simulink model "Controller_2_2_BangBang"  (R2019b)
settings: Solver=FixedStepAuto  StartTime=0.0  StopTime=Inf  FixedStep=0.0001  RelTol=1e-3  EnableMultiTasking=on
libraries: arduinolib x5, dspstat3 x2, simulink x1, powerlib_meascontrol x1
settings Model: SILPILModeSetting=veronly  ExtModeTrigDuration=2  Creator=mathe  LastModifiedBy=c3311409
settings OptimizationCC: EnhancedBackFolding=on  PassReuseOutputArgsAs=Individual arguments  ZeroExternalMemoryAtStartup=off  ZeroInternalMemoryAtStartup=off  MaxStackSize=64  OptimizeBlockOrder=speed  DifferentSizesBufferReuse=on  OptimizationCustomize=off  EfficientTunableParamExpr=on
settings DebuggingCC: ParameterTunabilityLossMsg=error
settings HardwareCC: ProdBitPerPointer=32  ProdBitPerSizeT=32  ProdBitPerPtrDiffT=32  ProdLargestAtomicInteger=Long  ProdLargestAtomicFloat=Double  ProdWordSize=32  ProdHWDeviceType=ARM Compatible->ARM Cortex
settings SFSimCC: MATLABDynamicMemAlloc=off
settings RTWCC: SystemTargetFile=ert.tlc  HardwareBoard=Arduino Due  TLCOptions=-aInlineSetEventsForThisBaseRateFcn=TLC_FALSE -aSuppressMultiTaskScheduler=TLC_FALSE -aRateBasedStepFcn=1  TemplateMakefile=ert_default_tmf  GenerateReport=on  Toolchain=Arduino ARM  BuildConfiguration=Faster Runs  IncludeHyperlinkInReport=on  LaunchReport=on  GenerateTraceInfo=on  GenerateTraceReport=on  GenerateTraceReportSl=on  GenerateTraceReportSf=on  GenerateTraceReportEml=on
settings CodeAppCC: ForceParamTrailComments=on  IgnoreCustomStorageClasses=off  OperatorAnnotations=on  SimulinkDataObjDesc=on  SFDataObjDesc=on  InsertBlockDesc=on
settings ERTTargetCC: SupportContinuousTime=on  SupportVariableSizeSignals=on  ExtModeStaticAllocSize=24576

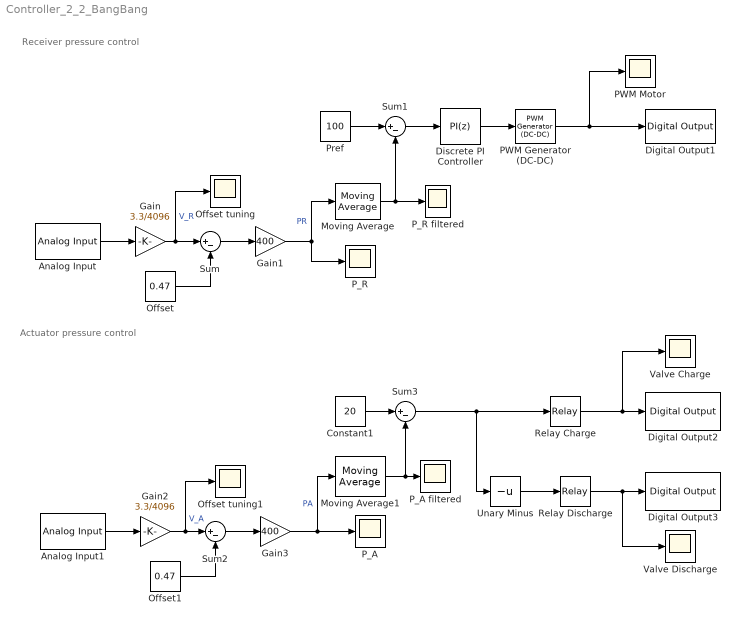
== system Controller_2_2_BangBang ==
  note: Actuator pressure control
  note: Receiver pressure control
  Analog Input : arduinolib/Analog Input  pinNumber=0  ReadResultsOnly=off  ConversionTriggerSource=Software  ExternalTriggerType=uint32(0)  OutputDataType=uint16  EnableConversionCompleteNotify=off  EnableOuputStatus=off  SampleTime=-1  blockPlatform=arduino
  Analog Input1 : arduinolib/Analog Input  pinNumber=1  ReadResultsOnly=off  ConversionTriggerSource=Software  ExternalTriggerType=uint32(0)  OutputDataType=uint16  EnableConversionCompleteNotify=off  EnableOuputStatus=off  SampleTime=-1  blockPlatform=arduino
  Constant1 : Constant  Value=20
  Digital Output1 : arduinolib/Digital Output  pinNumber=7  blockPlatform=arduino
  Digital Output2 : arduinolib/Digital Output  pinNumber=13  blockPlatform=arduino
  Digital Output3 : arduinolib/Digital Output  pinNumber=12  blockPlatform=arduino
  Discrete PI Controller : simulink/Continuous/PID Controller  Controller=PI  Form=Ideal  TimeDomain=Discrete-time  SampleTime=0.0001  IntegratorMethod=Trapezoidal  FilterMethod=Forward Euler  ControllerParametersSource=internal  P=0.001  I=10/(0.005*60)  D=0  UseFilter=on  N=100  TunerSelectOption=Transfer Function Based (PID Tuner App)  InitialConditionSource=internal  InitialConditionForIntegrator=0  InitialConditionForFilter=0  DifferentiatorICPrevScaledInput=0  ExternalReset=none  TrackingMode=off  Kt=1  LimitOutput=on  UpperSaturationLimit=1  LowerSaturationLimit=0  LinearizeAsGain=off  AntiWindupMode=clamping  Kb=1  POutMin=[]  POutMax=[]  IOutMin=[]  IOutMax=[]  DOutMin=[]  DOutMax=[]  NOutMin=[]  NOutMax=[]  SumOutMin=[]  SumOutMax=[]  SaturationOutMin=[]  SaturationOutMax=[]  PParamMin=[]  PParamMax=[]  IParamMin=[]  IParamMax=[]  DParamMin=[]  DParamMax=[]  NParamMin=[]  NParamMax=[]  KbParamMin=[]  KbParamMax=[]  KtParamMin=[]  KtParamMax=[]  KbOutMin=[]  KbOutMax=[]  KtOutMin=[]  KtOutMax=[]  IntegratorOutMin=[]  IntegratorOutMax=[]  FilterOutMin=[]  FilterOutMax=[]  SumI1OutMin=[]  SumI1OutMax=[]  SumI2OutMin=[]  SumI2OutMax=[]  SumI3OutMin=[]  SumI3OutMax=[]  SumI4OutMin=[]  SumI4OutMax=[]  SumDOutMin=[]  SumDOutMax=[]  DifferentiatorOutMin=[]  DifferentiatorOutMax=[]  FilterDiffOutCoefMin=[]  FilterDiffOutCoefMax=[]  ReciprocalOutMin=[]  ReciprocalOutMax=[]  SumDenOutMin=[]  SumDenOutMax=[]  SumNumOutMin=[]  SumNumOutMax=[]  DivideOutMin=[]  DivideOutMax=[]  IntegratorContinuousStateAttributes=''  IntegratorStateMustResolveToSignalObject=off  IntegratorRTWStateStorageClass=Auto  FilterContinuousStateAttributes=''  FilterStateMustResolveToSignalObject=off  FilterRTWStateStorageClass=Auto  ParallelPVariant=Passthrough  IdealPVariant=InternalParameters  IVariant=InternalParameters  DVariant=Disabled  IntegratorVariant=Discrete  SatVariant=Enabled  AWVariant=DiscClampingIdeal  PCopyVariant=InternalParamsIdeal  TRVariant=Disabled  FdbkBlocksVariant=Feedback  IdealPFdbkVariant=InternalParameters  SatFdbkVariant=Passthrough  DerivativeFilterVariant=Disabled  NVariant=Disabled  NCopyVariant=Disabled_SignalSpec  FilterICVariant=Disabled  IntegratorICVariant=InternalICs  ExternalResetVariant=Disabled  TRSumVariant=Passthrough  SumFdbkVariant=Enabled  SumVariant=Sum_PI
  Gain : Gain  Gain=3.3/4096
  Gain1 : Gain  Gain=400
  Gain2 : Gain  Gain=3.3/4096
  Gain3 : Gain  Gain=400
  Moving Average : dspstat3/Moving Average  Method=Sliding window  ForgettingFactorPort=off  SpecifyWindowLength=on  WindowLength=100  ForgettingFactor=0.9  SimulateUsing=Code generation
  Moving Average1 : dspstat3/Moving Average  Method=Sliding window  ForgettingFactorPort=off  SpecifyWindowLength=on  WindowLength=100  ForgettingFactor=0.9  SimulateUsing=Code generation
  Offset : Constant  Value=0.47
  Offset tuning : Scope
  Offset tuning1 : Scope
  Offset1 : Constant  Value=0.47
  PWM Generator (DC-DC) : powerlib_meascontrol/Pulse & Signal Generators/PWM Generator (DC-DC)  Fsw=4000  Ts=0.0001
      settings: SourceProductName=Simscape Electrical
  PWM Motor : Scope
  P_A : Scope
  P_A filtered : Scope
  P_R : Scope
  P_R filtered : Scope
  Pref : Constant  Value=100
  Relay Charge : Relay  OnSwitchValue=10  OffSwitchValue=0
  Relay Discharge : Relay  OnSwitchValue=10  OffSwitchValue=0
  Sum{,1..3} (4 alike) : Sum  Inputs=|+-
  Unary Minus : UnaryMinus
  Valve Charge : Scope
  Valve Discharge : Scope
  wires:
  Analog Input/1 -> Gain/1
  Gain/1 -> Offset tuning/1, Sum/1  "V_R"
  Offset/1 -> Sum/2
  Sum/1 -> Gain1/1
  Gain1/1 -> P_R/1, Moving Average/1  "PR"
  Pref/1 -> Sum1/1
  Sum1/1 -> Discrete PI Controller/1
  PWM Generator (DC-DC)/1 -> Digital Output1/1, PWM Motor/1
  Discrete PI Controller/1 -> PWM Generator (DC-DC)/1
  Moving Average/1 -> Sum1/2, P_R filtered/1
  Analog Input1/1 -> Gain2/1
  Offset1/1 -> Sum2/2
  Sum2/1 -> Gain3/1
  Gain2/1 -> Offset tuning1/1, Sum2/1  "V_A"
  Gain3/1 -> Moving Average1/1, P_A/1  "PA"
  Moving Average1/1 -> Sum3/2, P_A filtered/1
  Constant1/1 -> Sum3/1
  Relay Charge/1 -> Valve Charge/1, Digital Output2/1
  Sum3/1 -> Unary Minus/1, Relay Charge/1
  Relay Discharge/1 -> Valve Discharge/1, Digital Output3/1
  Unary Minus/1 -> Relay Discharge/1
